simulink model "limit_cycle_boost"  (R2018a)
settings: Solver=FixedStepAuto  StartTime=0.0  StopTime=1  FixedStep=Ti  RelTol=1e-3
undefined symbols (not defined in the file): Ad, Bd, Co, disturbance_Ro_enable, disturbance_Ro_time, disturbance_Vin_enable, disturbance_Vin_time, Ed, ell, Gd, Hd, kappa, L, opt_minimization, P, Qd, R, rho, Ro, Ro_p, sys, Ti, Ts, Vs, Vs_p, xe_h
libraries: powerlib x17, simulink x7
settings Model: SimulationMode=accelerator  Creator=TARCIO-FEM  LastModifiedBy=Julio-LEPO
settings OptimizationCC: EfficientMapNaN2IntZero=off
settings HardwareCC: TargetBitPerPointer=64  TargetBitPerSizeT=64  TargetBitPerPtrDiffT=64  TargetLongLongMode=on  TargetIntDivRoundTo=Zero  TargetEndianess=LittleEndian  TargetWordSize=64  TargetHWDeviceType=MATLAB Host  ProdEqTarget=off
settings CodeAppCC: MaxIdLength=128
settings GRTTargetCC: TargetLangStandard=C89/C90 (ANSI)  CombineOutputUpdateFcns=off  GRTInterface=on

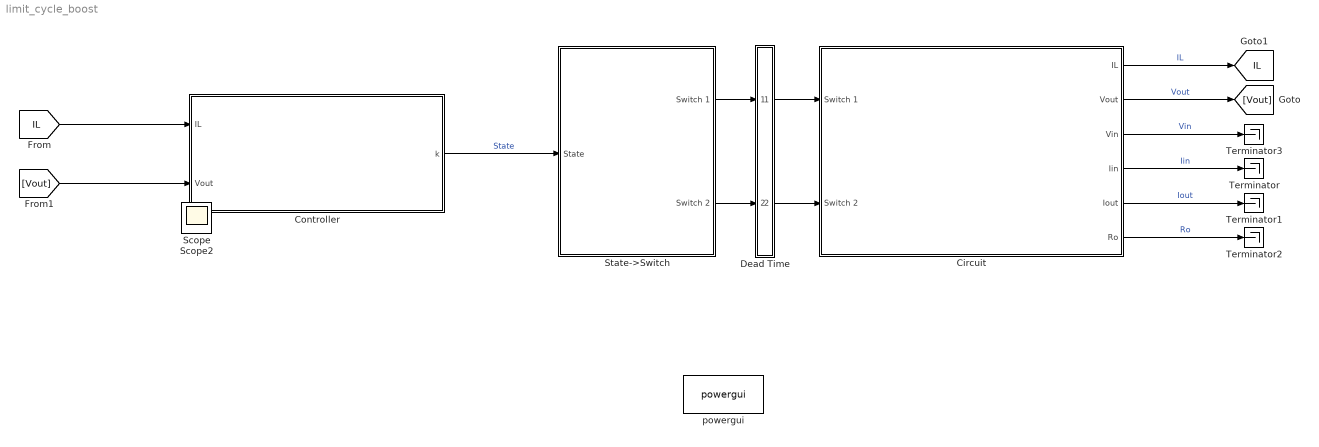
== system limit_cycle_boost ==
  Circuit : Subsystem
  Controller : Subsystem
  Dead Time : Subsystem
  State->Switch : Subsystem
  Terminator{,1..3} (4 alike) : Terminator
  powergui : powerlib/powergui  Priority=1  SimulationMode=Discrete  SampleTime=Ti  frequency=60  Iterations=50  frequencyindice=0  Pbase=100e6  ErrMax=1e-4  UnitsV=kV  UnitsW=MW  buscounter=0  FunctionMessages=off  echomessages=off  EnableUseOfTLC=off  CurrentSourceSwitches=off  DisableSnubberDevices=off  DisableRonSwitches=off  DisableVfSwitches=off  DisplayEquations=off  SolverType=Tustin/Backward Euler (TBE)  Interpol=off  ExternalGateDelay=off  methode=off  Ts=100  x0status=blocks  SPID=off  SwTol=0  HookPort=off  RestoreLinks=warning  ResistiveCurrentMeasurement=off  Frange=[0:2:500]  Ylog=off  Xlog=on  ShowGrid=off  save=off  variable=ZData  structure=0  ZoomFFT=off  StartTime=0.0  cycles=1  DisplayStyle=1  fundamental=60  FreqAxis=off  MaxFrequency=1000  frequencyindicesteady=1  RmsSteady=1  display=off
  Scope : Scope
  Scope2 : Scope
  tag scope: IL=global
  wires:
  Controller/1(k) -> State->Switch/1(State)  "State"
  [IL] -> Controller/1(IL)
  [Vout] -> Controller/2(Vout)
  Circuit/5(Iout) -> Terminator1/1  "Iout"
  Circuit/6(Ro) -> Terminator2/1  "Ro"
  Circuit/1(IL) -> [IL]  "IL"
  Circuit/4(Iin) -> Terminator/1  "Iin"
  Circuit/2(Vout) -> [Vout]  "Vout"
  Circuit/3(Vin) -> Terminator3/1  "Vin"
  State->Switch/2(Switch 2) -> Dead Time/2(In2)
  Dead Time/2(Out2) -> Circuit/2(Switch 2)
  State->Switch/1(Switch 1) -> Dead Time/1(In1)
  Dead Time/1(Out1) -> Circuit/1(Switch 1)

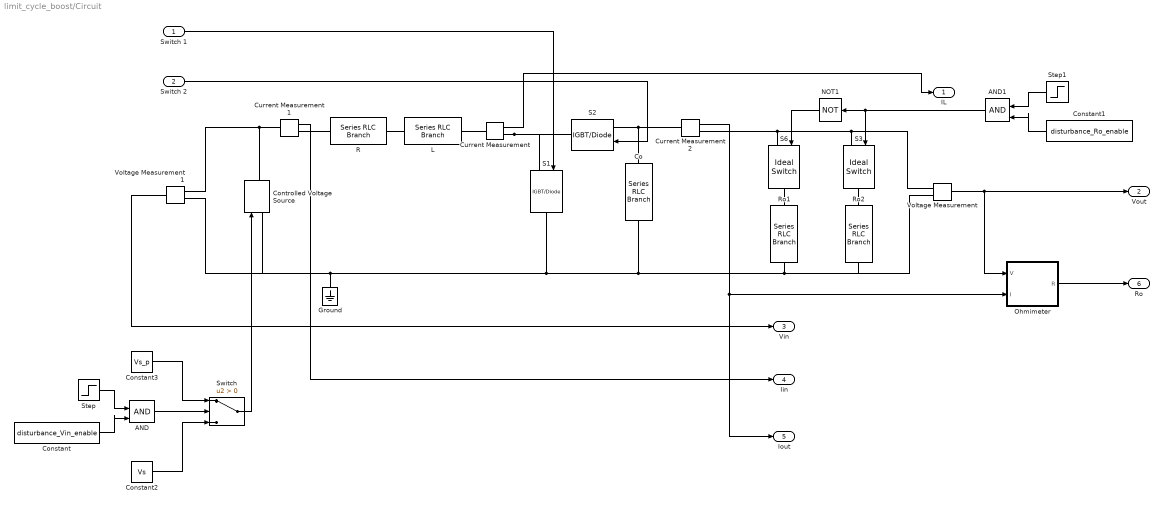
== system limit_cycle_boost/Circuit ==
  Switch 1 : Inport
  Switch 2 : Inport  Port=2
  AND : Logic  IconShape=distinctive  AllPortsSameDT=off  OutDataTypeStr=boolean
  AND1 : Logic  IconShape=distinctive  AllPortsSameDT=off  OutDataTypeStr=boolean
  Co : powerlib/Elements/Series RLC Branch  LConnTagsString=__new0  RConnTagsString=__new0  BranchType=C  Resistance=1  Inductance=L  SetiL0=off  InitialCurrent=0  Capacitance=Co  Setx0=on  InitialVoltage=Vs*Ro/(R+Ro)  Measurements=None
  Constant : Constant  Value=disturbance_Vin_enable
  Constant1 : Constant  Value=disturbance_Ro_enable
  Constant2 : Constant  Value=Vs
  Constant3 : Constant  Value=Vs_p
  Controlled Voltage Source : powerlib/Electrical Sources/Controlled Voltage Source  Initialize=on  Source_Type=DC  Amplitude=0  Phase=0  Frequency=0  Measurements=None
  Current Measurement : powerlib/Measurements/Current Measurement  PhasorSimulation=off  OutputType=Complex  PSBequivalent=0
  Current Measurement1 : powerlib/Measurements/Current Measurement  PhasorSimulation=off  OutputType=Complex  PSBequivalent=0
  Current Measurement2 : powerlib/Measurements/Current Measurement  PhasorSimulation=off  OutputType=Complex  PSBequivalent=0
  Ground : powerlib/Elements/Ground  LConnTagsString=a
  L : powerlib/Elements/Series RLC Branch  LConnTagsString=__new0  RConnTagsString=__new0  BranchType=L  Resistance=1  Inductance=L  SetiL0=off  InitialCurrent=0  Capacitance=1e-6  Setx0=off  InitialVoltage=0  Measurements=None
  NOT1 : Logic  Operator=NOT  IconShape=distinctive  AllPortsSameDT=off  OutDataTypeStr=boolean
  Ohmimeter : Subsystem
  R : powerlib/Elements/Series RLC Branch  LConnTagsString=__new0  RConnTagsString=__new0  BranchType=R  Resistance=R  Inductance=1e-3  SetiL0=off  InitialCurrent=0  Capacitance=1e-6  Setx0=off  InitialVoltage=0  Measurements=None
  Ro1 : powerlib/Elements/Series RLC Branch  LConnTagsString=__new0  RConnTagsString=__new0  BranchType=R  Resistance=Ro  Inductance=1e-3  SetiL0=off  InitialCurrent=0  Capacitance=1e-6  Setx0=off  InitialVoltage=0  Measurements=None
  Ro2 : powerlib/Elements/Series RLC Branch  LConnTagsString=__new0  RConnTagsString=__new0  BranchType=R  Resistance=Ro_p  Inductance=1e-3  SetiL0=off  InitialCurrent=0  Capacitance=1e-6  Setx0=off  InitialVoltage=0  Measurements=None
  S1 : powerlib/Power Electronics/IGBT//Diode  Ron=1e-3  Rs=1e5  Cs=inf  Measurements=off
  S2 : powerlib/Power Electronics/IGBT//Diode  Ron=1e-3  Rs=1e5  Cs=inf  Measurements=off
  S3 : powerlib/Power Electronics/Ideal Switch  Ron=0.001  Lon=0  IC=0  Rs=1e5  Cs=inf  Measurements=off
  S6 : powerlib/Power Electronics/Ideal Switch  Ron=0.001  Lon=0  IC=0  Rs=1e5  Cs=inf  Measurements=off
  Step : Step  Time=disturbance_Vin_time  SampleTime=0
  Step1 : Step  Time=disturbance_Ro_time  SampleTime=0
  Switch : Switch  Criteria=u2 > Threshold
  Voltage Measurement : powerlib/Measurements/Voltage Measurement  PhasorSimulation=off  OutputType=Complex  PSBequivalent=0
  Voltage Measurement1 : powerlib/Measurements/Voltage Measurement  PhasorSimulation=off  OutputType=Complex  PSBequivalent=0
  IL : Outport
  Vout : Outport  Port=2
  Vin : Outport  Port=3
  Iin : Outport  Port=4
  Iout : Outport  Port=5
  Ro : Outport  Port=6
  wires:
  Switch 1/1 -> S1/1
  Voltage Measurement1/1 -> Vin/1
  Current Measurement/1 -> IL/1
  Voltage Measurement/1 -> Vout/1, Ohmimeter/1(V)
  Switch 2/1 -> S2/1
  NOT1/1 -> S6/1
  Step/1 -> AND/1
  Constant/1 -> AND/2
  Step1/1 -> AND1/1
  Constant1/1 -> AND1/2
  AND1/1 -> S3/1, NOT1/1
  Switch/1 -> Controlled Voltage Source/1
  AND/1 -> Switch/2
  Constant3/1 -> Switch/1
  Constant2/1 -> Switch/3
  Current Measurement1/1 -> Iin/1
  Current Measurement2/1 -> Iout/1, Ohmimeter/2(I)
  Ohmimeter/1(R) -> Ro/1
  connections:
  L/LConn1 -- R/RConn1
  Current Measurement/LConn1 -- L/RConn1
  Controlled Voltage Source/RConn1 -- Current Measurement1/LConn1 -- Voltage Measurement1/LConn1
  S6/LConn1 -- Voltage Measurement/LConn1 -- S3/LConn1 -- Current Measurement2/RConn1
  Ro1/RConn1 -- Co/RConn1 -- S1/RConn1 -- Controlled Voltage Source/LConn1 -- Voltage Measurement1/LConn2 -- Ground/LConn1 -- Voltage Measurement/LConn2 -- Ro2/RConn1
  Current Measurement/RConn1 -- S2/RConn1 -- S1/LConn1
  S3/RConn1 -- Ro2/LConn1
  S6/RConn1 -- Ro1/LConn1
  Current Measurement1/RConn1 -- R/LConn1
  Current Measurement2/LConn1 -- S2/LConn1 -- Co/LConn1

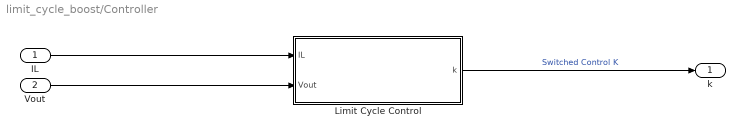
== system limit_cycle_boost/Controller ==
  IL : Inport
  Vout : Inport  Port=2
  Limit Cycle Control : Subsystem
  k : Outport
  wires:
  IL/1 -> Limit Cycle Control/1(IL)
  Vout/1 -> Limit Cycle Control/2(Vout)
  Limit Cycle Control/1(k) -> k/1  "Switched Control K"

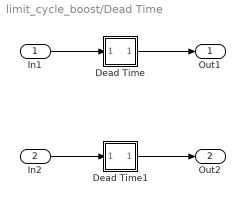
== system limit_cycle_boost/Dead Time ==
  In1 : Inport
  In2 : Inport  Port=2
  Dead Time : Subsystem
  Dead Time1 : Subsystem
  Out1 : Outport
  Out2 : Outport  Port=2
  wires:
  Dead Time1/1(Signal Delayed) -> Out2/1
  In1/1 -> Dead Time/1(Signal)
  Dead Time/1(Signal Delayed) -> Out1/1
  In2/1 -> Dead Time1/1(Signal)

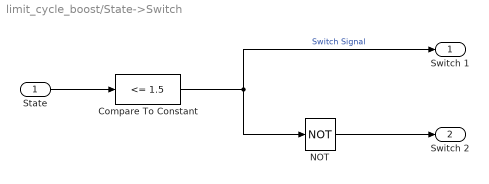
== system limit_cycle_boost/State->Switch ==
  State : Inport
  Compare To Constant : simulink/Logic and Bit Operations/Compare To Constant  relop=<=  const=1.5  OutDataTypeStr=boolean
  NOT : Logic  Operator=NOT  IconShape=distinctive  AllPortsSameDT=off  OutDataTypeStr=boolean
  Switch 1 : Outport
  Switch 2 : Outport  Port=2
  wires:
  Compare To Constant/1 -> Switch 1/1, NOT/1  "Switch Signal"
  State/1 -> Compare To Constant/1
  NOT/1 -> Switch 2/1

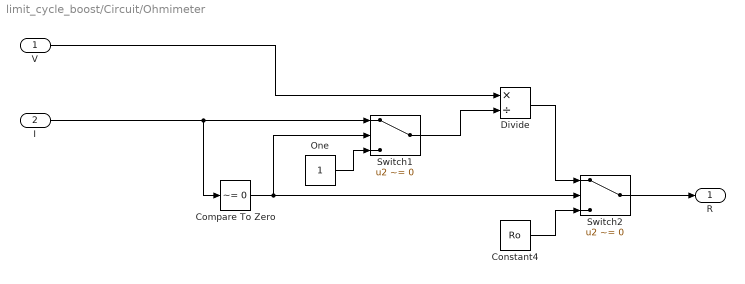
== system limit_cycle_boost/Circuit/Ohmimeter ==
  V : Inport
  I : Inport  Port=2
  Compare To Zero : simulink/Logic and Bit Operations/Compare To Zero  relop=~=  OutDataTypeStr=boolean
  Constant4 : Constant  Value=Ro
  Divide : Product  Inputs=*/
  One : Constant
  Switch1 : Switch  Criteria=u2 ~= 0
  Switch2 : Switch  Criteria=u2 ~= 0
  R : Outport
  wires:
  Compare To Zero/1 -> Switch1/2, Switch2/2
  I/1 -> Switch1/1, Compare To Zero/1
  Divide/1 -> Switch2/1
  Constant4/1 -> Switch2/3
  Switch1/1 -> Divide/2
  One/1 -> Switch1/3
  V/1 -> Divide/1
  Switch2/1 -> R/1

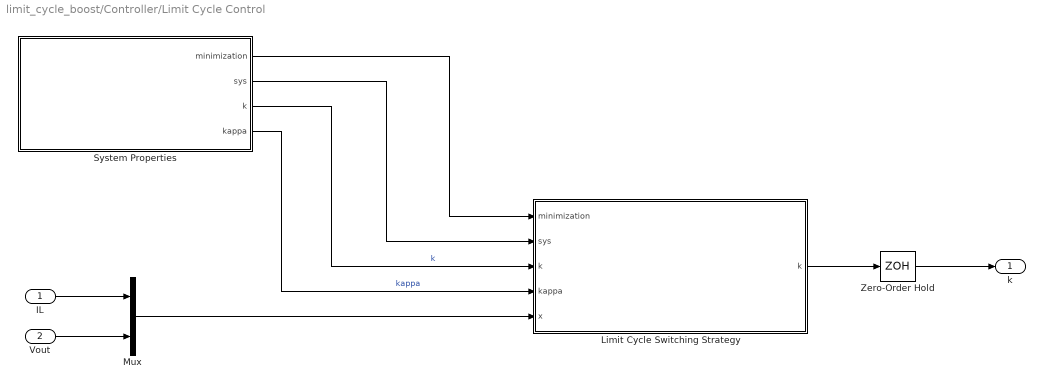
== system limit_cycle_boost/Controller/Limit Cycle Control ==
  IL : Inport
  Vout : Inport  Port=2
  Limit Cycle Switching Strategy : MATLAB Function  TreatAsAtomicUnit=on
  Mux : Mux  Inputs=2
  System Properties : Subsystem
  Zero-Order Hold : ZeroOrderHold  SampleTime=Ts
  k : Outport
  wires:
  Limit Cycle Switching Strategy/1(k) -> Zero-Order Hold/1
  System Properties/1(minimization) -> Limit Cycle Switching Strategy/1(minimization)
  System Properties/2(sys) -> Limit Cycle Switching Strategy/2(sys)
  Mux/1 -> Limit Cycle Switching Strategy/5(x)
  IL/1 -> Mux/1
  Vout/1 -> Mux/2
  Zero-Order Hold/1 -> k/1
  System Properties/3(k) -> Limit Cycle Switching Strategy/3("k ")  "k"
  System Properties/4(kappa) -> Limit Cycle Switching Strategy/4(kappa)  "kappa"

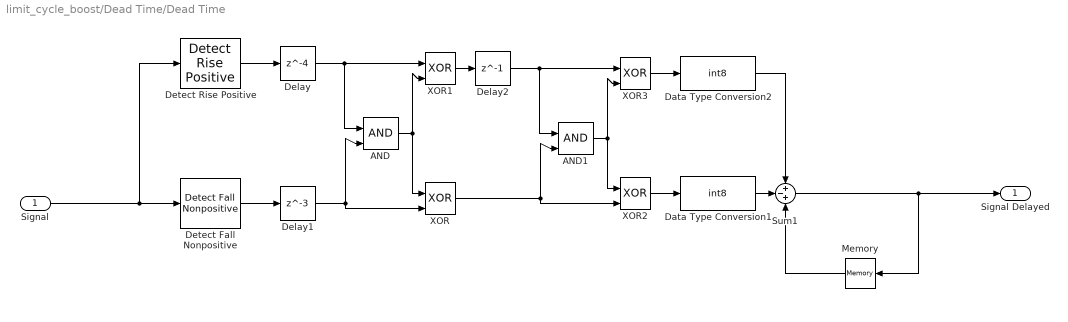
== system limit_cycle_boost/Dead Time/Dead Time ==
  Signal : Inport
  AND : Logic  IconShape=distinctive  AllPortsSameDT=off  OutDataTypeStr=boolean
  AND1 : Logic  IconShape=distinctive  AllPortsSameDT=off  OutDataTypeStr=boolean
  Data Type Conversion1 : DataTypeConversion  OutDataTypeStr=int8
  Data Type Conversion2 : DataTypeConversion  OutDataTypeStr=int8
  Delay : Delay  DelayLength=4
  Delay1 : Delay  DelayLength=3
  Delay2 : Delay  DelayLength=1
  Detect Fall Nonpositive : simulink/Logic and Bit Operations/Detect Fall Nonpositive  vinit=0  OutDataTypeStr=boolean
      settings: SourceProductName=Simulink  SourceProductBaseCode=SL
  Detect Rise Positive : simulink/Logic and Bit Operations/Detect Rise Positive  vinit=0  OutDataTypeStr=boolean
  Memory : Memory  InheritSampleTime=on  LinearizeAsDelay=on
  Sum1 : Sum  Inputs=+-+
  XOR{,1..3} (4 alike) : Logic  Operator=XOR  IconShape=distinctive  AllPortsSameDT=off  OutDataTypeStr=boolean
  Signal Delayed : Outport
  wires:
  Sum1/1 -> Memory/1, Signal Delayed/1
  Data Type Conversion1/1 -> Sum1/2
  Memory/1 -> Sum1/3
  Signal/1 -> Detect Rise Positive/1, Detect Fall Nonpositive/1
  Data Type Conversion2/1 -> Sum1/1
  Detect Fall Nonpositive/1 -> Delay1/1
  Detect Rise Positive/1 -> Delay/1
  Delay1/1 -> XOR/2, AND/2
  Delay/1 -> XOR1/1, AND/1
  XOR1/1 -> Delay2/1
  AND/1 -> XOR1/2, XOR/1
  Delay2/1 -> XOR3/1, AND1/1
  AND1/1 -> XOR3/2, XOR2/1
  XOR/1 -> XOR2/2, AND1/2
  XOR3/1 -> Data Type Conversion2/1
  XOR2/1 -> Data Type Conversion1/1

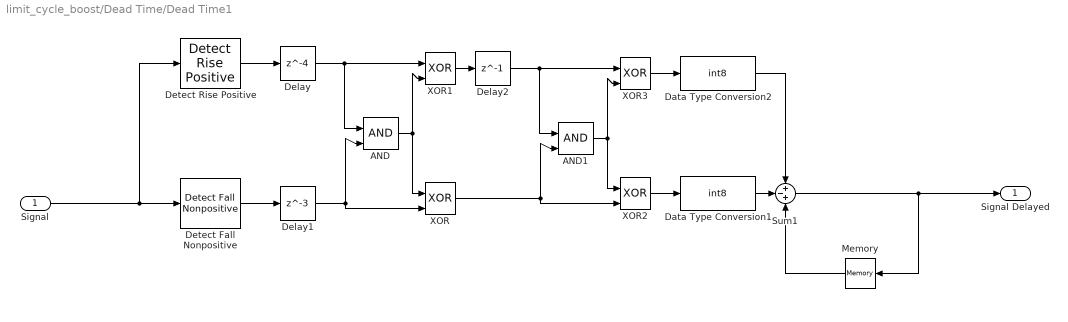
== system limit_cycle_boost/Dead Time/Dead Time1 ==
  Signal : Inport
  AND : Logic  IconShape=distinctive  AllPortsSameDT=off  OutDataTypeStr=boolean
  AND1 : Logic  IconShape=distinctive  AllPortsSameDT=off  OutDataTypeStr=boolean
  Data Type Conversion1 : DataTypeConversion  OutDataTypeStr=int8
  Data Type Conversion2 : DataTypeConversion  OutDataTypeStr=int8
  Delay : Delay  DelayLength=4
  Delay1 : Delay  DelayLength=3
  Delay2 : Delay  DelayLength=1
  Detect Fall Nonpositive : simulink/Logic and Bit Operations/Detect Fall Nonpositive  vinit=0  OutDataTypeStr=boolean
      settings: SourceProductName=Simulink  SourceProductBaseCode=SL
  Detect Rise Positive : simulink/Logic and Bit Operations/Detect Rise Positive  vinit=0  OutDataTypeStr=boolean
  Memory : Memory  InheritSampleTime=on  LinearizeAsDelay=on
  Sum1 : Sum  Inputs=+-+
  XOR{,1..3} (4 alike) : Logic  Operator=XOR  IconShape=distinctive  AllPortsSameDT=off  OutDataTypeStr=boolean
  Signal Delayed : Outport
  wires:
  Sum1/1 -> Memory/1, Signal Delayed/1
  Data Type Conversion1/1 -> Sum1/2
  Memory/1 -> Sum1/3
  Signal/1 -> Detect Rise Positive/1, Detect Fall Nonpositive/1
  Data Type Conversion2/1 -> Sum1/1
  Detect Fall Nonpositive/1 -> Delay1/1
  Detect Rise Positive/1 -> Delay/1
  Delay1/1 -> XOR/2, AND/2
  Delay/1 -> XOR1/1, AND/1
  XOR1/1 -> Delay2/1
  AND/1 -> XOR1/2, XOR/1
  Delay2/1 -> XOR3/1, AND1/1
  AND1/1 -> XOR3/2, XOR2/1
  XOR/1 -> XOR2/2, AND1/2
  XOR3/1 -> Data Type Conversion2/1
  XOR2/1 -> Data Type Conversion1/1

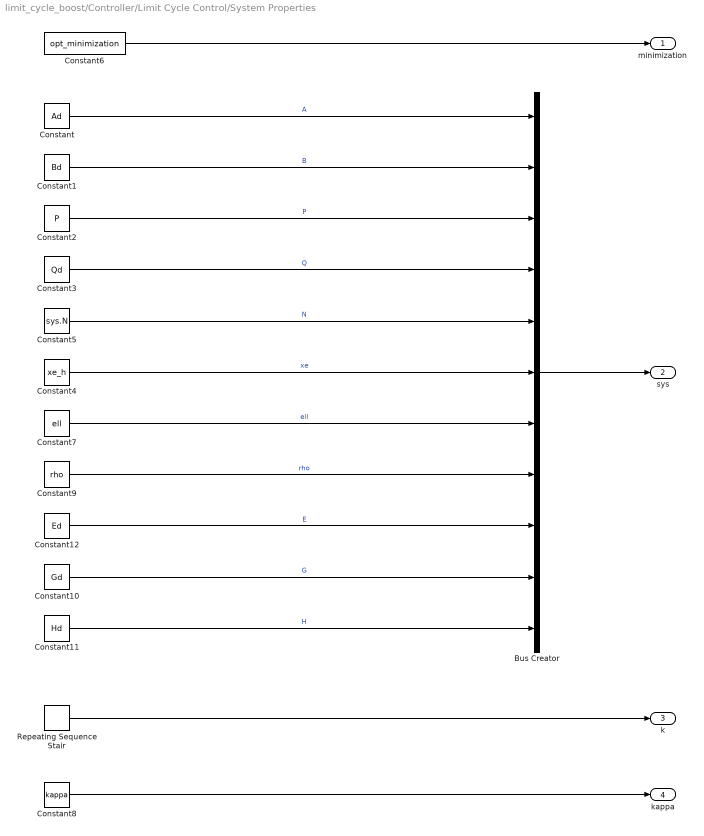
== system limit_cycle_boost/Controller/Limit Cycle Control/System Properties ==
  Bus Creator : BusCreator  Inputs=11  OutDataTypeStr=Bus: SystemDataBus
  Constant : Constant  Value=Ad  VectorParams1D=off
  Constant1 : Constant  Value=Bd  VectorParams1D=off
  Constant10 : Constant  Value=Gd  VectorParams1D=off
  Constant11 : Constant  Value=Hd  VectorParams1D=off
  Constant12 : Constant  Value=Ed  VectorParams1D=off
  Constant2 : Constant  Value=P  VectorParams1D=off
  Constant3 : Constant  Value=Qd  VectorParams1D=off
  Constant4 : Constant  Value=xe_h  VectorParams1D=off
  Constant5 : Constant  Value=sys.N
  Constant6 : Constant  Value=opt_minimization
  Constant7 : Constant  Value=ell  VectorParams1D=off
  Constant8 : Constant  Value=kappa
  Constant9 : Constant  Value=rho  VectorParams1D=off
  Repeating Sequence Stair : simulink/Sources/Repeating Sequence Stair  OutValues=[1:kappa].'  tsamp=Ts  OutMin=[]  OutMax=[]  OutDataTypeStr=double  OutputDataTypeScalingMode=double  OutDataType=fixdt(0,8)  ConRadixGroup=Best Precision: Vector-wise  OutScaling=2^-12
  minimization : Outport
  sys : Outport  Port=2
  k : Outport  Port=3
  kappa : Outport  Port=4
  wires:
  Bus Creator/1 -> sys/1
  Constant2/1 -> Bus Creator/3  "P"
  Constant1/1 -> Bus Creator/2  "B"
  Constant/1 -> Bus Creator/1  "A"
  Constant3/1 -> Bus Creator/4  "Q"
  Constant5/1 -> Bus Creator/5  "N"
  Constant6/1 -> minimization/1
  Constant4/1 -> Bus Creator/6  "xe"
  Constant7/1 -> Bus Creator/7  "ell"
  Repeating Sequence Stair/1 -> k/1
  Constant8/1 -> kappa/1
  Constant9/1 -> Bus Creator/8  "rho"
  Constant11/1 -> Bus Creator/11  "H"
  Constant10/1 -> Bus Creator/10  "G"
  Constant12/1 -> Bus Creator/9  "E"

== matlab function limit_cycle_boost/Controller/Limit Cycle Control/Limit Cycle Switching Strategy ==
  data: minimization input; sys input; k input; kappa input; x input; k output
function k = discrete_switching_strategy(minimization, sys, k, kappa, x)
    
    km = mod(k, kappa)+1;
    
    A = sys.A;
    Q = sys.Q;
    E = sys.E;
    G = sys.G;
    H = sys.H;
    xe = sys.xe(:,k);
    P = sys.P(:,:,km);
    Pk = sys.P(:,:,k);
    ell = sys.ell;
    rho = sys.rho;
    
    Xi = x - xe;
    
    sig = zeros(sys.N,1);
    
    for i=1:sys.N
        switch(minimization)
            case 1
                sig(i) = [Xi;1]'*[
                    A(:,:,i)'*P*A(:,:,i)-Pk+E(:,:,i)'*E(:,:,i)  A(:,:,i)'*P*ell(:,k,i)
                    ell(:,k,i)'*P*A(:,:,i)                      ell(:,k,i)'*P*ell(:,k,i)
                    ]*[Xi;1];
            case 2
                sig(i) = [Xi;1]'*[
                    A(:,:,i)'*P*A(:,:,i)-Pk+E(:,:,i)'*E(:,:,i)  A(:,:,i)'*P*ell(:,k,i)
                    ell(:,k,i)'*P*A(:,:,i)                      ell(:,k,i)'*P*ell(:,k,i)
                    ]*[Xi;1];
            case 3
                Lcal = [
                        A(:,:,i)'*P*A(:,:,i)-Pk      A(:,:,i)'*P*ell(:,k,i)
                        ell(:,k,i)'*P*A(:,:,i)        ell(:,k,i)'*P*ell(:,k,i)
                        ];
                Dcal = [A(:,:,i)'*P*H(:,:,i)+E(:,:,i)'*G(:,:,i);
                        ell(:,k,i)'*P*H(:,:,i)];
                Sigmacal = H(:,:,i)'*P*H(:,:,i)+G(:,:,i)'*G(:,:,i)-rho*eye(size(H(:,:,i),2));
                Mcal=Dcal/Sigmacal*Dcal';
                sig(i) = [Xi;1]'*(Lcal-Mcal)*[Xi;1]-(Xi)'*Q(:,:,i)*(Xi);
        end
    end
    [~, k] = min(sig);
end
